simulink model "ode45vdp"  (R2017a)
settings: Solver=VariableStepAuto  StartTime=0.0  StopTime=20  RelTol=1e-3
settings Model: Creator=eruffaldi  LastModifiedBy=eruffaldi

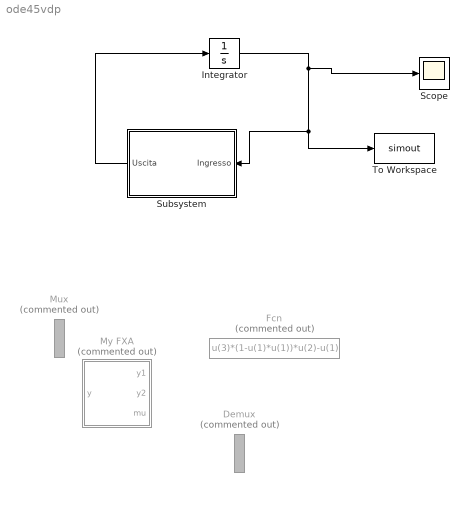
== system ode45vdp ==
  Demux : Demux  Commented=on  Outputs=2
  Fcn : Fcn  Commented=on  Expr=u(3)*(1-u(1)*u(1))*u(2)-u(1)
  Integrator : Integrator  InitialCondition=[2,0]
  Mux : Mux  Commented=on  Inputs=2
  My FXA : MATLAB Function  Commented=on  TreatAsAtomicUnit=on
  Scope : Scope
  Subsystem : Subsystem  mask{mu=57.0}
      mask prompts: mu "Mu Value"
  To Workspace : ToWorkspace  VariableName=simout  SaveFormat=Timeseries  SampleTime=-1
  wires:
  Integrator/1 -> Scope/1, Subsystem/1(Ingresso), To Workspace/1
  Subsystem/1(Uscita) -> Integrator/1

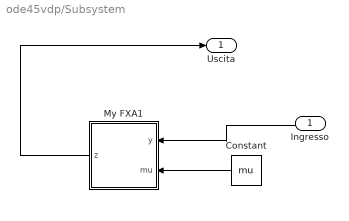
== system ode45vdp/Subsystem ==
  Ingresso : Inport
  Constant : Constant  Value=mu
  My FXA1 : MATLAB Function  TreatAsAtomicUnit=on
  Uscita : Outport
  wires:
  My FXA1/1(z) -> Uscita/1
  Ingresso/1 -> My FXA1/1(y)
  Constant/1 -> My FXA1/2(mu)

== matlab function ode45vdp/Subsystem/My FXA1 ==
  data: y input; z output; mu input
function z = fcn(y,mu)

z = [y(2); mu*(1-y(1)^2)*y(2)-y(1)];

== matlab function ode45vdp/My FXA ==
  data: y1 input; y output; y2 input; mu input
function y = fcn(y1,y2,mu)

y = mu*(1-y1^2)*y2-y1;
